simulink model "Model_StimulationTherapy"  (R2024a)
settings: Solver=FixedStepAuto  StartTime=0.0  StopTime=inf  RelTol=1e-3
settings Model: PauseTimes=1  Creator=Javi  LastModifiedBy=Pedaleo FES
settings SolverCC: AlgebraicLoopSolver=TrustRegion
settings DataIOCC: ReturnWorkspaceOutputs=off
settings OptimizationCC: ReuseModelBlockBuffer=off  LifeSpan=inf
settings DebuggingCC: UnconnectedInputMsg=warning  UnconnectedOutputMsg=warning  UnconnectedLineMsg=warning  ArithmeticOperatorsInVariantConditions=warning
settings ModelReferenceCC: EnableRefExpFcnMdlSchedulingChecks=on
settings SFSimCC: SimUseLocalCustomCode=off  CustomCodeUndefinedFunction=UseInterfaceOnly
settings RTWCC: RTWUseLocalCustomCode=off  BuildConfiguration=Faster Runs  GPUComputeCapability=3.5
settings CodeAppCC: StateflowObjectComments=on

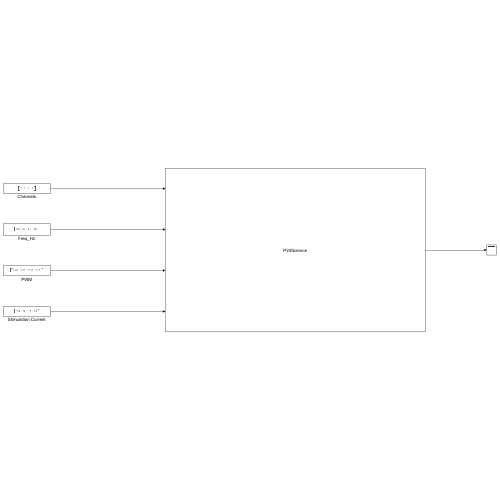
[thumbnail: Simulink's stored preview of the top-level diagram]
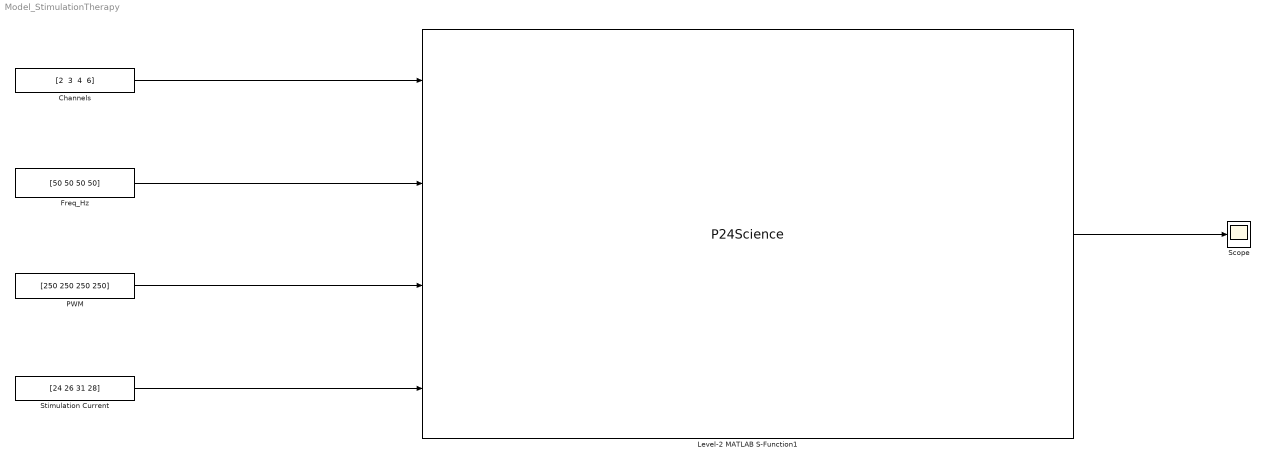
== system Model_StimulationTherapy ==
  Channels : Constant  Value="[2  3  4  6]"
  Freq_Hz : Constant  Value=[50 50 50 50]
  Level-2 MATLAB S-Function1 : M-S-Function  FunctionName=P24Science
  PWM : Constant  Value=[250 250 250 250]
  Scope : Scope
  Stimulation Current : Constant  Value=[24 26 31 28]
  wires:
  PWM/1 -> Level-2 MATLAB S-Function1/3
  Channels/1 -> Level-2 MATLAB S-Function1/1
  Freq_Hz/1 -> Level-2 MATLAB S-Function1/2
  Stimulation Current/1 -> Level-2 MATLAB S-Function1/4
  Level-2 MATLAB S-Function1/1 -> Scope/1
